simulink model "eventCameraUAVDemo"  (R2023a)
settings: Solver=FixedStepDiscrete  StartTime=0.0  StopTime=10  FixedStep=1/30  RelTol=1e-3
StopFcn:
  | if evalin('base', 'exist(''eventLog'', ''var'')'), s = struct('eventLog', evalin('base', 'eventLog')); eventCameraSummary(s); end
undefined symbols (not defined in the file or in its folder): Sim3dSensor
libraries: eventcameralib x4, sim3dlib x3
Description:
  | Event camera (DVS) simulation of a UAV city flyover using Sim 3D. Demonstrates the EventCamera, EventVisualizer, and eventCameraSummary workflow.
settings Model: Creator=csaunder  LastModifiedBy=csaunder
settings DebuggingCC: UnconnectedInputMsg=warning  UnconnectedOutputMsg=warning  UnconnectedLineMsg=warning
settings ModelReferenceCC: UpdateModelReferenceTargets=IfOutOfDate
settings RTWCC: GPUComputeCapability=5.0
settings GRTTargetCC: SupportVariableSizeSignals=on
settings ConfigComp: CovBoundaryAbsTol=1.0e-5

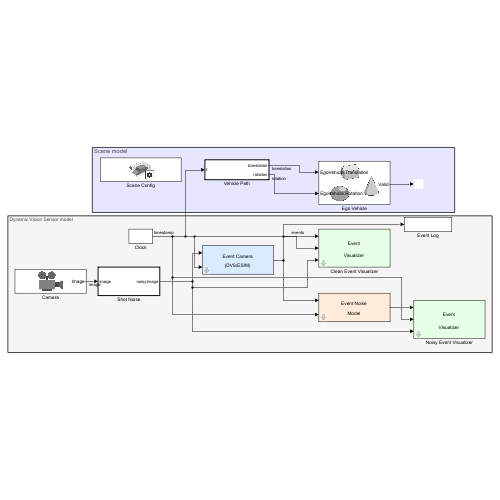
[thumbnail: Simulink's stored preview of the top-level diagram]
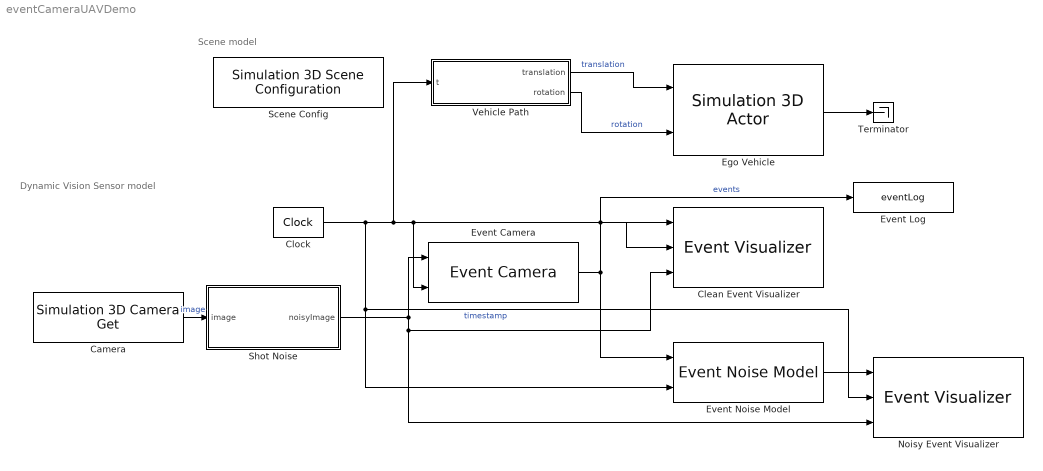
== system eventCameraUAVDemo ==
  note: Dynamic Vision Sensor model
  note: Scene model
  Camera : sim3dlib/Simulation 3D Camera Get  Priority=1  sensorTag=Sim3dSensor�  sensorId=1  sensorName=Sim3dSensor�  vehTagList={'Scene Origin', 'EgoVehicle'}  vehTag=EgoVehicle  CoordinateSystem=Default  mountLoc=Origin  offsetFlag=on  tmountOffset=[0 0 0]  rmountOffset=[0 0 0]  HorizontalResolution=320  VerticalResolution=240  HorizontalFOV=90  SampleTime=1/30  mountPoint=[0 0 0]  mountOrientation=[0 0 0]  aMode=aMode  ID=1
  Clean Event Visualizer : eventcameralib/Event Visualizer  ImageHeight=240  ImageWidth=320  TimeSurfaceDecay=0.3
      settings: SourceProductName=Event Camera
  Clock : DigitalClock  SampleTime=1/30
  Ego Vehicle : sim3dlib/Simulation 3D Actor  Priority=1  ActorName=EgoVehicle  ParentName=Scene Origin  Operation=Create at setup  InitScriptText=|  SampleTime=1/30  Translation=[25 0 20]  Rotation=[0 0 0]  Scale=[1 1 1]  InputsText=EgoVehicle.Translation EgoVehicle.Rotation  aMode=aMode  ActorTag=EgoVehicle  ActorType=Sim3dActor  ID=C
      | % Reserved keywords:
      | % - Actor : handle to this actor object
      | % - World : handle to the world object
      | 
      | % Examples:
      | 
      | % Create a primitive geometry (optional)
      | % createShape(Actor, 'box', [1 1 1]);
      | 
      | % Initialize values (optional)
      | % Actor.Physics = true;
      | % Actor.Color = [1 0 0];
  Event Camera : eventcameralib/Event Camera  ContrastThresholdOn=0.2  ContrastThresholdOff=0.2  MaxEventsPerFrame=500000  RefractoryPeriod=0  BandwidthHz=Inf  ThresholdMismatch=0  PixelLatency=100e-6
      settings: SourceProductName=Event Camera
  Event Log : ToWorkspace  VariableName=eventLog  SaveFormat=Timeseries  SampleTime=-1
  Event Noise Model : eventcameralib/Event Noise Model  ImageHeight=240  ImageWidth=320  BackgroundRate=100  TimestampJitter=50e-6  NumHotPixels=5  HotPixelRate=1000  LeakRate=0  MaxEventsPerStep=500000
      settings: SourceProductName=Event Camera
  Noisy Event Visualizer : eventcameralib/Event Visualizer  ImageHeight=240  ImageWidth=320  TimeSurfaceDecay=0.3
      settings: SourceProductName=Event Camera
  Scene Config : sim3dlib/Simulation 3D Scene Configuration  Priority=0  ProjectFormat=Default Scenes  SceneDesc=US city block  ProjectName=C:\Program Files\MATLAB\R2026a\toolbox\shared\sim3d_projects\automotive_project_windows\UE\WindowsNoEditor\VehicleSimulation.exe  ScenePath=/Game/Maps/HwStrght  EnableOpenDRIVE=off  vehTagList={'Custom','Scene Origin','EgoVehicle'}  vehTag=EgoVehicle  FreeCameraDefaultInitialTranslation=[-6, 0, 2]  FreeCameraDefaultInitialRotation=[0, -15, 0]  FreeCameraInitialTranslation=[0 0 0]  FreeCameraInitialRotation=[0 0 0]  OpVisEn=off  Ts=1/30  EnableWindow=on  EnableRemoteAccess=off  SimulationMode=CoSimulation  SimulateUsing=Interpreted execution  EnableAnimationRecording=off  OverrideDefaultRecording=off  AnimationRecordingFileName=sim3dAnimation.mat  AnimationRecordingInterval=[0 inf]  EnableWeather=off  SunAzimuth=90  SunAltitude=40.0  wind=1  clouds=10  fog=0  rain=0  EnableGeospatial=off  UseTrueOrigin=off  OriginHeight=200  OriginLatitude=40.744652  OriginLongitude=-73.988864  MapStyle=Aerial  AdditionalAssetIDs=[]  UseAdvancedSunSky=off  SolarTime=11  TimeZone=-5  Day=21  Month=9  Year=2022  UseDaylightSavingTime=on  DSTStartDay=10  DSTStartMonth=3  DSTEndDay=3  DSTEndMonth=11  DSTSwitchHour=2  sensorTag=MainCamera1  sensorId=1  sensorName=MainCamera1  mountLoc=Origin  offsetFlag=off  tmountOffset=[0, 0, 0]  rmountOffset=[0, 0, 0]  HorizontalResolution=1280  VerticalResolution=720  HorizontalFOV=60  mountPoint=[0 0 0]  mountOrientation=[0 0 0]  aMode=aMode  ID=1  GeoTrigger=Inactive
  Shot Noise : MATLAB Function  TreatAsAtomicUnit=on
  Terminator : Terminator
  Vehicle Path : MATLAB Function  TreatAsAtomicUnit=on
  wires:
  Camera/1 -> Shot Noise/1(image)  "image"
  Shot Noise/1(noisyImage) -> Clean Event Visualizer/3, Noisy Event Visualizer/3, Event Camera/1
  Clock/1 -> Clean Event Visualizer/2, Event Camera/2, Vehicle Path/1(t), Noisy Event Visualizer/2, Event Noise Model/2  "timestamp"
  Event Camera/1 -> Clean Event Visualizer/1, Event Log/1, Event Noise Model/1  "events"
  Event Noise Model/1 -> Noisy Event Visualizer/1
  Vehicle Path/1(translation) -> Ego Vehicle/1  "translation"
  Vehicle Path/2(rotation) -> Ego Vehicle/2  "rotation"
  Ego Vehicle/1 -> Terminator/1

== matlab function eventCameraUAVDemo/Vehicle Path ==
  data: t input; translation output; rotation output
function [translation, rotation] = vehiclePath(t)
% UAV flying through city at 8 m/s, 25m altitude, turning a corner
% Smooth 90-degree left turn using a circular arc
speed = 8;
altitude = 20;
xOffset = 25;       % starting position offset (m)
turnStart = 3;      % begin turn at t=4s
turnRadius = 20;    % radius of turn (m)
turnArc = pi/2;     % 90 degrees
turnDuration = turnRadius * turnArc / speed;  % time to complete arc
turnEnd = turnStart + turnDuration;

if t < turnStart
    % Straight segment along +X
    x = xOffset + speed * t;
    y = 0;
    yaw = 0;
elseif t < turnEnd
    % Circular arc turning left (toward +Y)
    arcDist = speed * (t - turnStart);
    theta = arcDist / turnRadius;
    xEntry = xOffset + speed * turnStart;
    x = xEntry + turnRadius * sin(theta);
    y = turnRadius * (1 - cos(theta));
    yaw = theta;  % radians
else
    % Straight segment along +Y after turn
    xEntry = xOffset + speed * turnStart;
    x = xEntry + turnRadius;
    y = turnRadius + speed * (t - turnEnd);
    yaw = pi/2;
end

translation = [x, y, altitude];
rotation = [0, 0, yaw];  % [Roll, Pitch, Yaw] in radians
end

== matlab function eventCameraUAVDemo/Shot Noise ==
  data: image input; noisyImage output
function noisyImage = shotNoise(image)
%#codegen
% Simulate photon shot noise by scaling to approximate photon counts,
% applying Poisson sampling, then scaling back.
exposureGain = 5000; % approximate photon count at full white
im01 = double(image) / 255;
photons = im01 * exposureGain;
noisy = poissrnd(photons);
noisyImage = uint8(min(noisy / exposureGain * 255, 255));
